simulink model "DSSS_Two_Channels"  (R2017a)
settings: Solver=VariableStepAuto  StartTime=0.0  StopTime=10  RelTol=1e-3
libraries: commutil2 x9, commdigbbndpm3 x3, commsink2 x2, commseqgen3 x2, commfilt2 x2, commrandsrc3 x2
settings Model: Creator=rooki  LastModifiedBy=rooki

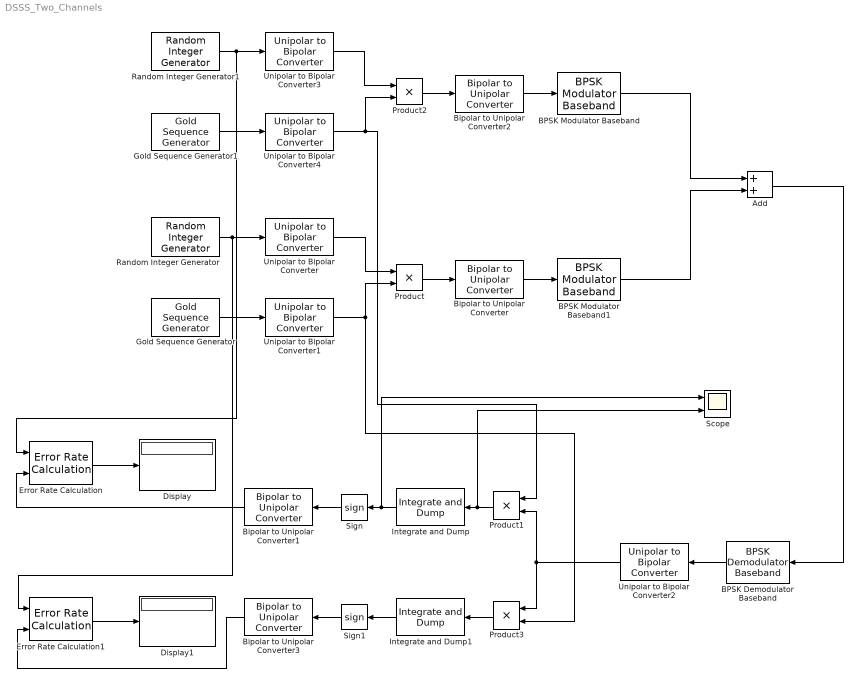
== system DSSS_Two_Channels ==
  Add : Sum
  BPSK Demodulator Baseband : commdigbbndpm3/BPSK Demodulator Baseband  DecType=Hard decision  VarSource=Dialog  Variance=1  Ph=0  outDtype=Inherit via internal rule  derotateFactorWordLen=16  derotateFactorDataTypeStr=Inherit: Same word length as input  derotateFactorLastDataTypeStr=Inherit: Same word length as input
  BPSK Modulator Baseband : commdigbbndpm3/BPSK Modulator Baseband  Ph=0  outDtype=double  outWordLen=16  outUDDataType=sfix(16)  outFracLenMode=Best precision  outFracLen=15  outDataTypeStr=double  outLastDataTypeStr=double
  BPSK Modulator Baseband1 : commdigbbndpm3/BPSK Modulator Baseband  Ph=0  outDtype=double  outWordLen=16  outUDDataType=sfix(16)  outFracLenMode=Best precision  outFracLen=15  outDataTypeStr=double  outLastDataTypeStr=double
  Bipolar to Unipolar Converter{,1..3} (4 alike) : commutil2/Bipolar to Unipolar Converter  M=2  polarity=Positive  dataType=Inherit via internal rule
      settings: SourceProductName=Communications System Toolbox  SourceProductBaseCode=CM
  Display : Display
  Display1 : Display
  Error Rate Calculation : commsink2/Error Rate Calculation  N=1  st_delay=0  cp_mode=Entire frame  subframe=[]  PMode=Port  WsName=ErrorVec  RsMode2=off  stop=off  numErr=100  maxBits=1e6
  Error Rate Calculation1 : commsink2/Error Rate Calculation  N=1  st_delay=0  cp_mode=Entire frame  subframe=[]  PMode=Port  WsName=ErrorVec  RsMode2=off  stop=off  numErr=100  maxBits=1e6
  Gold Sequence Generator : commseqgen3/Gold Sequence Generator  genPoly1='z^6 + z + 1'  iniState1=[0 0 0 0 0 1]  genPoly2='z^6 + z^5 + z^2 + z + 1'  iniState2=[0 0 0 0 0 1]  index=0  shift=0  outVarSiz=off  maxOutSizeMode=Dialog parameter  maxOutSize=[10 1]  Ts=1/32000  sampPerFrame=1  reset=off  outDataType=double
      settings: SourceProductName=Communications System Toolbox  SourceProductBaseCode=CM
  Gold Sequence Generator1 : commseqgen3/Gold Sequence Generator  genPoly1='z^6 + z + 1'  iniState1=[1 0 0 1 0 0]  genPoly2='z^6 + z^5 + z^2 + z + 1'  iniState2=[1 0 0 1 0 0]  index=0  shift=0  outVarSiz=off  maxOutSizeMode=Dialog parameter  maxOutSize=[10 1]  Ts=1/32000  sampPerFrame=1  reset=off  outDataType=double
      settings: SourceProductName=Communications System Toolbox  SourceProductBaseCode=CM
  Integrate and Dump : commfilt2/Integrate and Dump  obssamples=32  offsetsamples=0  nodump=off  roundingMode=Floor  overflowMode=off  outputDataTypeStr=Inherit: Same as accumulator  outputLastDataTypeStr=Inherit: Same as accumulator
      settings: SourceProductName=Communications System Toolbox
  Integrate and Dump1 : commfilt2/Integrate and Dump  obssamples=32  offsetsamples=0  nodump=off  roundingMode=Floor  overflowMode=off  outputDataTypeStr=Inherit: Same as accumulator  outputLastDataTypeStr=Inherit: Same as accumulator
      settings: SourceProductName=Communications System Toolbox
  Product{,1..3} (4 alike) : Product
  Random Integer Generator : commrandsrc3/Random Integer Generator  SetSize=2  SeedSource=Parameter  Seed=3453  SampleTime=1/1000  SamplesPerFrame=1  OutputDataType=double  SimulateUsing=Interpreted execution
  Random Integer Generator1 : commrandsrc3/Random Integer Generator  SetSize=2  SeedSource=Parameter  Seed=33  SampleTime=1/1000  SamplesPerFrame=1  OutputDataType=double  SimulateUsing=Interpreted execution
  Scope : Scope  NumInputPorts=2
  Sign : Signum
  Sign1 : Signum
  Unipolar to Bipolar Converter{,1..4} (5 alike) : commutil2/Unipolar to Bipolar Converter  M=2  polarity=Positive  dataType=Inherit via internal rule
      settings: SourceProductName=Communications System Toolbox
  wires:
  Random Integer Generator/1 -> Error Rate Calculation1/1, Unipolar to Bipolar Converter/1
  Gold Sequence Generator/1 -> Unipolar to Bipolar Converter1/1
  Unipolar to Bipolar Converter/1 -> Product/1
  Unipolar to Bipolar Converter1/1 -> Product3/2, Product/2
  Product/1 -> Bipolar to Unipolar Converter/1
  Error Rate Calculation/1 -> Display/1
  Product1/1 -> Scope/2, Integrate and Dump/1
  Add/1 -> BPSK Demodulator Baseband/1
  BPSK Demodulator Baseband/1 -> Unipolar to Bipolar Converter2/1
  Unipolar to Bipolar Converter2/1 -> Product1/2, Product3/1
  Integrate and Dump/1 -> Scope/1, Sign/1
  Sign/1 -> Bipolar to Unipolar Converter1/1
  Bipolar to Unipolar Converter1/1 -> Error Rate Calculation/2
  Random Integer Generator1/1 -> Unipolar to Bipolar Converter3/1, Error Rate Calculation/1
  Unipolar to Bipolar Converter3/1 -> Product2/1
  Product2/1 -> Bipolar to Unipolar Converter2/1
  Gold Sequence Generator1/1 -> Unipolar to Bipolar Converter4/1
  Product3/1 -> Integrate and Dump1/1
  Sign1/1 -> Bipolar to Unipolar Converter3/1
  Integrate and Dump1/1 -> Sign1/1
  Error Rate Calculation1/1 -> Display1/1
  Bipolar to Unipolar Converter3/1 -> Error Rate Calculation1/2
  Bipolar to Unipolar Converter2/1 -> BPSK Modulator Baseband/1
  Bipolar to Unipolar Converter/1 -> BPSK Modulator Baseband1/1
  BPSK Modulator Baseband/1 -> Add/1
  BPSK Modulator Baseband1/1 -> Add/2
  Unipolar to Bipolar Converter4/1 -> Product1/1, Product2/2
